simulink model "Speed_control_of_three_phase_SCIM"  (R2021b)
settings: Solver=VariableStepAuto  StartTime=0.0  StopTime=1.0  RelTol=1e-3
libraries: spsIGBTLib x6, simulink x3, spsAsynchronousMachinepuUnitsLib x1, spsDCVoltageSourceLib x1, spsGroundLib x1, spsSawtoothGeneratorLib x1, spsThreePhaseParallelRLCBranchLib x1, spsThreePhaseVIMeasurementLib x1, spspowerguiLib x1
settings Model: Creator=mluser  LastModifiedBy=Soham Kundu

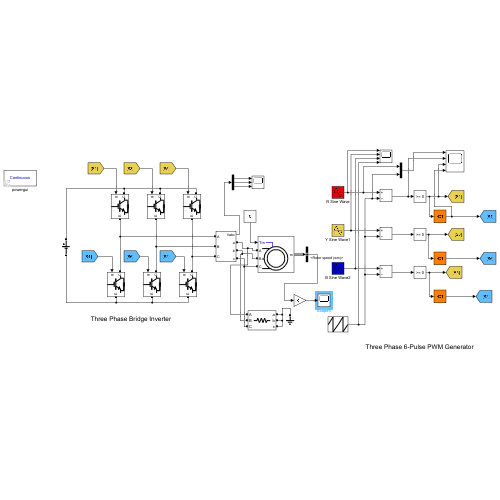
[thumbnail: Simulink's stored preview of the top-level diagram]
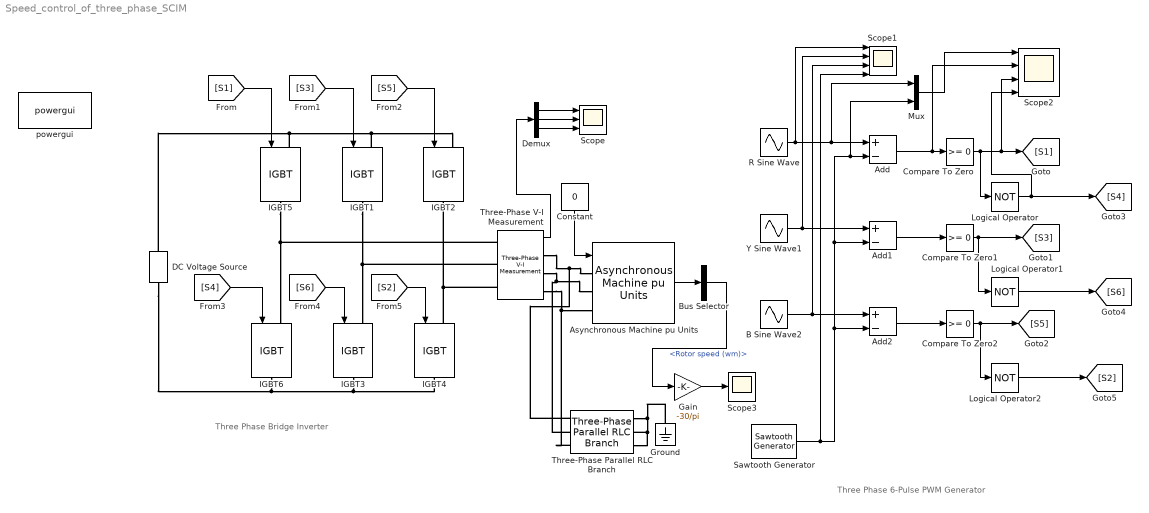
== system Speed_control_of_three_phase_SCIM ==
  note: Three Phase 6-Pulse PWM Generator
  note: Three Phase Bridge Inverter
  Add : Sum  Inputs=+-
  Add1 : Sum  Inputs=+-
  Add2 : Sum  Inputs=+-
  Asynchronous Machine pu Units : spsAsynchronousMachinepuUnitsLib/Asynchronous Machine pu Units  RotorType=Squirrel-cage  PresetModel=No  MechanicalLoad=Torque Tm  ShowDetailedParameters=on  ReferenceFrame=Rotor  Units=pu  MeasurementBus=off  NominalParameters=[3730 460 60]  VoltageRatio=1  Stator=[0.01965 0.0397]  Rotor=[0.01909 0.0397]  Cage1=[0.01909 0.0397]  Cage2=[0.01909 0.0397]  Lm=1.354  Mechanical=[0.09526 0.05479 2]  PolePairs=2  InitialConditions="[ 1,0   0,0,0   0,0,0 ]"  SimulateSaturation=off  Saturation="[0.212,0.4201,0.8125,1.0979,1.4799,2.2457,3.2586,4.5763,6.4763 ;   0.5,0.7,0.9,1,1.1,1.2 ,1.3,1.4,1.5]"  LoadFlowParameters=0  TsPowergui=0  TsBlock=-1  IterativeModel=Trapezoidal non iterative  IterativeDiscreteModel=Trapezoidal non iterative  Pmec=0
      settings: SourceProductBaseCode=PS
  B Sine Wave2 : Sin  Frequency=2*pi*50  Phase=-2*pi/3  SampleTime=0
  Bus Selector : BusSelector  OutputSignals=Mechanical.Rotor speed (wm)
  Compare To Zero : simulink/Logic and Bit Operations/Compare To Zero  relop=>=  OutDataTypeStr=boolean
  Compare To Zero1 : simulink/Logic and Bit Operations/Compare To Zero  relop=>=  OutDataTypeStr=boolean
  Compare To Zero2 : simulink/Logic and Bit Operations/Compare To Zero  relop=>=  OutDataTypeStr=boolean
  Constant : Constant  Value=0
  DC Voltage Source : spsDCVoltageSourceLib/DC Voltage Source  Amplitude=100  Measurements=None
  Demux : Demux  Outputs=3
  Gain : Gain  Gain=-30/pi
  Ground : spsGroundLib/Ground  LConnTagsString=a
  IGBT{1..6} (6 alike) : spsIGBTLib/IGBT  Ron=0.001  Lon=0  Vf=1  Tf=1e-6  Tt=2e-6  IC=0  Rs=1e5  Cs=inf  Measurements=off
  Logical Operator : Logic  Operator=NOT  AllPortsSameDT=off  OutDataTypeStr=boolean
  Logical Operator1 : Logic  Operator=NOT  AllPortsSameDT=off  OutDataTypeStr=boolean
  Logical Operator2 : Logic  Operator=NOT  AllPortsSameDT=off  OutDataTypeStr=boolean
  Mux : Mux  Inputs=2
  R Sine Wave : Sin  Frequency=2*pi*50  SampleTime=0
  Sawtooth Generator : spsSawtoothGeneratorLib/Sawtooth Generator  Freq=600  Phase=180  Ts=0
  Scope : Scope  NumInputPorts=3
  Scope1 : Scope  NumInputPorts=4
  Scope2 : Scope  NumInputPorts=4
  Scope3 : Scope
  Three-Phase Parallel RLC Branch : spsThreePhaseParallelRLCBranchLib/Three-Phase Parallel RLC Branch  LConnTagsString=A|B|C  RConnTagsString=A|B|C  BranchType=R  Resistance=1  Inductance=1e-3  Capacitance=1e-6  Measurements=None
      settings: SourceProductBaseCode=PS
  Three-Phase V-I Measurement : spsThreePhaseVIMeasurementLib/Three-Phase V-I Measurement  VoltageMeasurement=phase-to-ground  SetLabelV=off  LabelV=Vabc  Vpu=off  VpuLL=off  CurrentMeasurement=no  SetLabelI=off  LabelI=Iabc  Ipu=off  Pbase=100e6  Vbase=500e3  OutputType=Complex  PhasorSimulation=off  PSBequivalent=0
  Y Sine Wave1 : Sin  Frequency=2*pi*50  Phase=2*pi/3  SampleTime=0
  powergui : spspowerguiLib/powergui  Priority=1  SimulationMode=Continuous  SampleTime=50e-6  frequency=60  Iterations=50  frequencyindice=0  Pbase=100e6  ErrMax=1e-4  UnitsV=kV  UnitsW=MW  buscounter=0  FunctionMessages=off  echomessages=off  EnableUseOfTLC=off  CurrentSourceSwitches=off  DisableSnubberDevices=off  DisableRonSwitches=off  DisableVfSwitches=off  DisplayEquations=off  AutomaticDiscreteSolvers=off  SolverType=Tustin/Backward Euler (TBE)  Interpol=off  ExternalGateDelay=off  methode=off  Ts=100  x0status=blocks  SPID=on  SwTol=0  HookPort=off  NonlinearTolerance=1e-4  nMaxIteration=100  ContinueOnMaxIteration=off  RestoreLinks=warning  ResistiveCurrentMeasurement=off  Frange=[0:2:500]  Ylog=off  Xlog=on  ShowGrid=off  save=off  variable=ZData  structure=0  ZoomFFT=off  StartTime=0.0  cycles=1  DisplayStyle=1  fundamental=60  FreqAxis=off  MaxFrequency=1000  frequencyindicesteady=1  RmsSteady=1  display=off
  wires:
  R Sine Wave/1 -> Scope1/1, Mux/1, Add/1
  Y Sine Wave1/1 -> Scope1/2, Add1/1
  B Sine Wave2/1 -> Scope1/3, Add2/1
  Sawtooth Generator/1 -> Scope1/4, Add2/2, Add1/2, Mux/2, Add/2
  Add/1 -> Scope2/2, Compare To Zero/1
  Add1/1 -> Compare To Zero1/1
  Add2/1 -> Compare To Zero2/1
  Compare To Zero/1 -> Logical Operator/1, Scope2/3, [S1]
  Compare To Zero1/1 -> Logical Operator1/1, [S3]
  Compare To Zero2/1 -> Logical Operator2/1, [S5]
  Logical Operator/1 -> Scope2/4, [S4]
  Logical Operator1/1 -> [S6]
  Logical Operator2/1 -> [S2]
  [S1] -> IGBT5/1
  [S5] -> IGBT2/1
  [S3] -> IGBT1/1
  [S4] -> IGBT6/1
  [S6] -> IGBT3/1
  [S2] -> IGBT4/1
  Three-Phase V-I Measurement/1 -> Demux/1
  Demux/1 -> Scope/1
  Demux/2 -> Scope/2
  Demux/3 -> Scope/3
  Mux/1 -> Scope2/1
  Constant/1 -> Asynchronous Machine pu Units/1
  Gain/1 -> Scope3/1
  Asynchronous Machine pu Units/1 -> Bus Selector/1
  Bus Selector/1 -> Gain/1  "<Rotor speed (wm)>"
  connections:
  IGBT4/LConn1 -- Three-Phase V-I Measurement/LConn3 -- IGBT2/RConn1
  IGBT1/RConn1 -- IGBT3/LConn1 -- Three-Phase V-I Measurement/LConn2
  IGBT5/RConn1 -- IGBT6/LConn1 -- Three-Phase V-I Measurement/LConn1
  DC Voltage Source/RConn1 -- IGBT5/LConn1 -- IGBT1/LConn1 -- IGBT2/LConn1
  DC Voltage Source/LConn1 -- IGBT6/RConn1 -- IGBT3/RConn1 -- IGBT4/RConn1
  Three-Phase V-I Measurement/RConn1 -- Three-Phase Parallel RLC Branch/LConn1 -- Asynchronous Machine pu Units/LConn1
  Three-Phase V-I Measurement/RConn2 -- Three-Phase Parallel RLC Branch/LConn2 -- Asynchronous Machine pu Units/LConn2
  Three-Phase V-I Measurement/RConn3 -- Three-Phase Parallel RLC Branch/LConn3 -- Asynchronous Machine pu Units/LConn3
  Three-Phase Parallel RLC Branch/RConn1 -- Three-Phase Parallel RLC Branch/RConn3 -- Three-Phase Parallel RLC Branch/RConn2 -- Ground/LConn1
